simulink model "BatteryPack_calculation"  (R2024a)
settings: Solver=VariableStepAuto  StartTime=0.0  StopTime=10.0  RelTol=1e-3
settings Model: LastModifiedBy=Sai Vivek
settings RTWCC: GPUComputeCapability=3.5

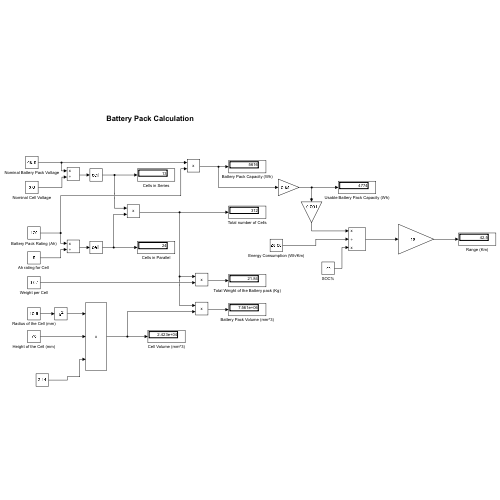
[thumbnail: Simulink's stored preview of the top-level diagram]
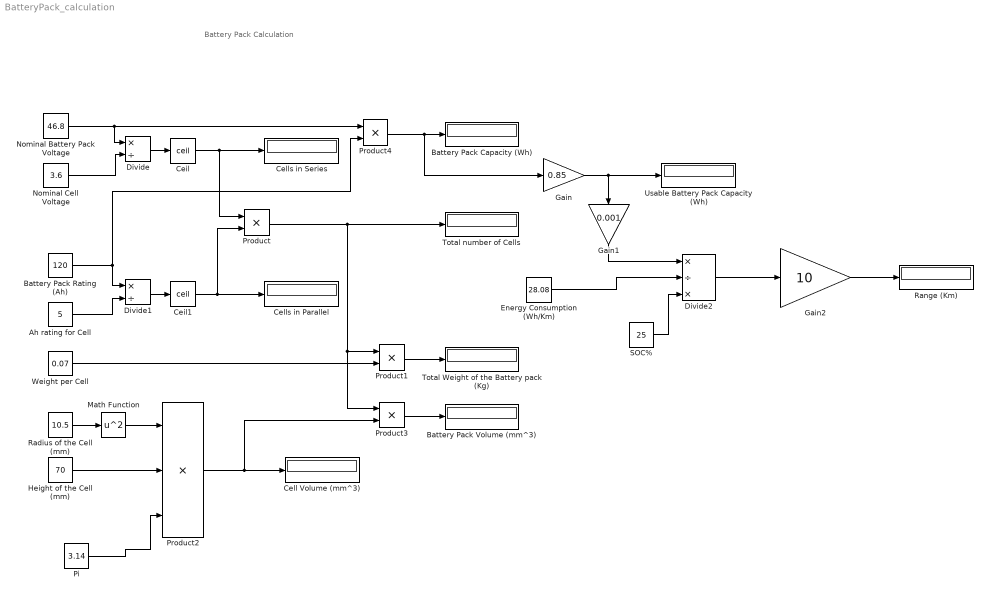
== system BatteryPack_calculation ==
  note: Battery Pack Calculation
  "Ah rating for Cell " : Constant  Value=5
  Battery Pack Capacity (Wh) : Display
  Battery Pack Rating (Ah) : Constant  Value=120
  Battery Pack Volume (mm^3) : Display
  Ceil : Rounding  Operator=ceil
  Ceil1 : Rounding  Operator=ceil
  Cell Volume (mm^3) : Display
  Cells in Parallel : Display
  Cells in Series : Display
  Divide : Product  Inputs=*/
  Divide1 : Product  Inputs=*/
  Divide2 : Product  Inputs=*/*
  Energy Consumption (Wh/Km) : Constant  Value=28.08
  Gain : Gain  Gain=0.85
  Gain1 : Gain  Gain=0.001
  Gain2 : Gain  Gain=10
  Height of the Cell (mm) : Constant  Value=70
  Math Function : Math  Operator=square
  Nominal Battery Pack Voltage : Constant  Value=46.8
  Nominal Cell Voltage : Constant  Value=3.6
  Pi : Constant  Value=3.14  OutDataTypeStr=Inherit: Inherit via back propagation
  Product{,1,3..4} (4 alike) : Product
  Product2 : Product  Inputs=3
  Radius of the Cell (mm) : Constant  Value=10.5
  Range (Km) : Display
  SOC% : Constant  Value=25
  Total Weight of the Battery pack (Kg) : Display
  Total number of Cells : Display
  Usable Battery Pack Capacity (Wh) : Display
  Weight per Cell : Constant  Value=0.07
  wires:
  Nominal Battery Pack Voltage/1 -> Product4/1, Divide/1
  Nominal Cell Voltage/1 -> Divide/2
  Battery Pack Rating (Ah)/1 -> Product4/2, Divide1/1
  "Ah rating for Cell "/1 -> Divide1/2
  Divide/1 -> Ceil/1
  Divide1/1 -> Ceil1/1
  Ceil/1 -> Product/1, Cells in Series/1
  Ceil1/1 -> Product/2, Cells in Parallel/1
  Weight per Cell/1 -> Product1/2
  Product/1 -> Product3/1, Product1/1, Total number of Cells/1
  Product1/1 -> Total Weight of the Battery pack (Kg)/1
  Pi/1 -> Product2/3
  Radius of the Cell (mm)/1 -> Math Function/1
  Math Function/1 -> Product2/1
  Height of the Cell (mm)/1 -> Product2/2
  Product2/1 -> Product3/2, Cell Volume (mm^3)/1
  Product3/1 -> Battery Pack Volume (mm^3)/1
  Product4/1 -> Gain/1, Battery Pack Capacity (Wh)/1
  Gain/1 -> Usable Battery Pack Capacity (Wh)/1, Gain1/1
  Energy Consumption (Wh/Km)/1 -> Divide2/2
  Divide2/1 -> Gain2/1
  Gain1/1 -> Divide2/1
  SOC%/1 -> Divide2/3
  Gain2/1 -> Range (Km)/1
